simulink model "agc"  (R2017a)
settings: Solver=VariableStepAuto  StartTime=0.0  StopTime=20  MaxStep=0.2  RelTol=1e-3
settings Model: Creator=Jon  LastModifiedBy=Jon

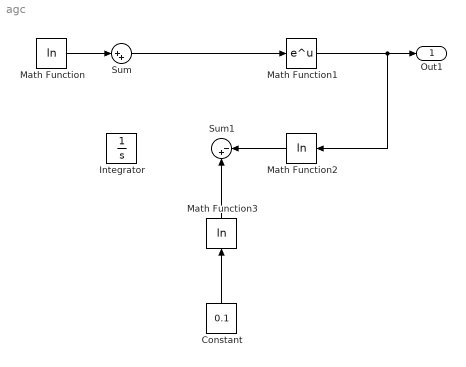
== system agc ==
  Constant : Constant  Value=0.1
  Integrator : Integrator
  Math Function : Math  Operator=log  SaturateOnIntegerOverflow=on
  Math Function1 : Math  SaturateOnIntegerOverflow=on
  Math Function2 : Math  Operator=log  SaturateOnIntegerOverflow=on
  Math Function3 : Math  Operator=log  SaturateOnIntegerOverflow=on
  Sum : Sum  Inputs=|++
  Sum1 : Sum  Inputs=|-+
  Out1 : Outport
  wires:
  Math Function/1 -> Sum/1
  Sum/1 -> Math Function1/1
  Math Function2/1 -> Sum1/1
  Math Function3/1 -> Sum1/2
  Constant/1 -> Math Function3/1
  Math Function1/1 -> Math Function2/1, Out1/1
